simulink model "VCMGCM1962020b_v2"  (R2020b)
settings: Solver=FixedStepDiscrete  StartTime=0.0  StopTime=10.0  FixedStep=0.005  RelTol=1e-3  EnableMultiTasking=on
PreLoadFcn:
  | try, model_open; catch, disp('Error occurred while executing model pre-load callback: model_open.m'); disp('Please assure that the MATLAB working directory is set to the model directory before opening.'); end
InitFcn:
  | try, model_open; catch, end
undefined symbols (not defined in the file): Bridge, GCM, H, raptor_get_param_eval, raptor_get_safe_string, raptor_xcp_function
libraries: Blocks_lib x1165, Raptor_lib x665, simulink x62, VCM_lib x5
(part 3 of 23)

== system VCMGCM1962020b_v2/Fgnd/Actuators/CAN/CCS Interface ==
  Data : Inport
  Bus Creator : BusCreator  Inputs=1
  CCSEV_ChargeParameters1 : Subsystem
      mask help:
      | Example of how to set up a CAN message transmit.
      | 1. Copy this block into the main model.
      | 2. Disable/break library link.
      | 3. Underneath, set up CAN Tx Message block.
      | 4. For each field, connect a CANTxField block from the CAN block to the bus creator; adjust parameters as necessary.
      mask init:
      | [msgnam, msgbus] = CANBlockInit('Tx');
      mask Display: disp(['CAN Tx: Message\n' msgnam '\n' msgbus]);
  CCSEV_ChargeParameters2 : Subsystem
      mask help:
      | Example of how to set up a CAN message transmit.
      | 1. Copy this block into the main model.
      | 2. Disable/break library link.
      | 3. Underneath, set up CAN Tx Message block.
      | 4. For each field, connect a CANTxField block from the CAN block to the bus creator; adjust parameters as necessary.
      mask init:
      | [msgnam, msgbus] = CANBlockInit('Tx');
      mask Display: disp(['CAN Tx: Message\n' msgnam '\n' msgbus]);
  CCSEV_DC_ChargeInfo1 : Subsystem
      mask help:
      | Example of how to set up a CAN message transmit.
      | 1. Copy this block into the main model.
      | 2. Disable/break library link.
      | 3. Underneath, set up CAN Tx Message block.
      | 4. For each field, connect a CANTxField block from the CAN block to the bus creator; adjust parameters as necessary.
      mask init:
      | [msgnam, msgbus] = CANBlockInit('Tx');
      mask Display: disp(['CAN Tx: Message\n' msgnam '\n' msgbus]);
  Commands : Subsystem
  Header : Blocks_lib/Header  width=Portrait  addtext=''
  MsgName : Subsystem
      mask help:
      | Example of how to set up a CAN message transmit.
      | 1. Copy this block into the main model.
      | 2. Disable/break library link.
      | 3. Underneath, set up CAN Tx Message block.
      | 4. For each field, connect a CANTxField block from the CAN block to the bus creator; adjust parameters as necessary.
      mask init:
      | [msgnam, msgbus] = CANBlockInit('Tx');
      mask Display: disp(['CAN Tx: Message\n' msgnam '\n' msgbus]);
  Act : Outport  VectorParamsAs1DForOutWhenUnconnected=off
  wires:
  Commands/1(Cmds) -> Bus Creator/1, MsgName/2(Cmd), CCSEV_DC_ChargeInfo1/2(Cmd)
  Data/1 -> CCSEV_DC_ChargeInfo1/1(Data), CCSEV_ChargeParameters2/1(Data), CCSEV_ChargeParameters1/1(Data), MsgName/1(Data), Commands/1(Data)
  Bus Creator/1 -> Act/1  "CCS"

== system VCMGCM1962020b_v2/Fgnd/Actuators/CAN/Charger ==
  Data : Inport
  ChgrBMSA : Subsystem
      mask help:
      | Example of how to set up a CAN message transmit.
      | 1. Copy this block into the main model.
      | 2. Disable/break library link.
      | 3. Underneath, set up CAN Tx Message block.
      | 4. For each field, connect a CANTxField block from the CAN block to the bus creator; adjust parameters as necessary.
      mask init:
      | [msgnam, msgbus] = CANBlockInit('Tx');
      mask Display: disp(['CAN Tx: Message\n' msgnam '\n' msgbus]);
  Config Msgs : Subsystem  Commented=on
  Ground : Ground
  Header : Blocks_lib/Header  width=Portrait  addtext=''
  Act : Outport  VectorParamsAs1DForOutWhenUnconnected=off
  wires:
  Data/1 -> ChgrBMSA/1(Data)
  Ground/1 -> Act/1  "Chgr"

== system VCMGCM1962020b_v2/Fgnd/Actuators/CAN/DC//DC Converter ==
  Data : Inport
  Ground : Ground
  Header : Blocks_lib/Header  width=Portrait  addtext=''
  MsgName : Subsystem
      mask help:
      | Example of how to set up a CAN message transmit.
      | 1. Copy this block into the main model.
      | 2. Disable/break library link.
      | 3. Underneath, set up CAN Tx Message block.
      | 4. For each field, connect a CANTxField block from the CAN block to the bus creator; adjust parameters as necessary.
      mask init:
      | [msgnam, msgbus] = CANBlockInit('Tx');
      mask Display: disp(['CAN Tx: Message\n' msgnam '\n' msgbus]);
  Act : Outport  VectorParamsAs1DForOutWhenUnconnected=off
  wires:
  Ground/1 -> Act/1  "DCDC"
  Data/1 -> MsgName/1(Data)

== system VCMGCM1962020b_v2/Fgnd/Actuators/CAN/DC//DC Converter1 ==
  Data : Inport
  DCDCDCDC_Cmmd_0_16V : Subsystem
      mask help:
      | Example of how to set up a CAN message transmit.
      | 1. Copy this block into the main model.
      | 2. Disable/break library link.
      | 3. Underneath, set up CAN Tx Message block.
      | 4. For each field, connect a CANTxField block from the CAN block to the bus creator; adjust parameters as necessary.
      mask init:
      | [msgnam, msgbus] = CANBlockInit('Tx');
      mask Display: disp(['CAN Tx: Message\n' msgnam '\n' msgbus]);
  Ground : Ground
  Header : Blocks_lib/Header  width=Portrait  addtext=''
  Act : Outport  VectorParamsAs1DForOutWhenUnconnected=off
  wires:
  Ground/1 -> Act/1  "DCDC"
  Data/1 -> DCDCDCDC_Cmmd_0_16V/1(Data)

== system VCMGCM1962020b_v2/Fgnd/Actuators/CAN/Display ==
  Data : Inport
  DisplayHVES1_D2 : Subsystem
      mask help:
      | Example of how to set up a CAN message transmit.
      | 1. Copy this block into the main model.
      | 2. Disable/break library link.
      | 3. Underneath, set up CAN Tx Message block.
      | 4. For each field, connect a CANTxField block from the CAN block to the bus creator; adjust parameters as necessary.
      mask init:
      | [msgnam, msgbus] = CANBlockInit('Tx');
      mask Display: disp(['CAN Tx: Message\n' msgnam '\n' msgbus]);
  Ground : Ground
  Header : Blocks_lib/Header  width=Portrait  addtext=''
  Act : Outport  VectorParamsAs1DForOutWhenUnconnected=off
  wires:
  Ground/1 -> Act/1  "Dspl"
  Data/1 -> DisplayHVES1_D2/1(Data)

== system VCMGCM1962020b_v2/Fgnd/Actuators/CAN/Drive Inverter ==
  Data : Inport
  Bus Creator : BusCreator  Inputs=1
  Bus Selector : BusSelector  OutputSignals=Sensors.CAN.DrvInvtr.EM1.EM1MsgVld [Bool],Control.Mode.StartStop.RunMode [Bool]
  Bus Selector1 : BusSelector  OutputSignals=Sensors.CAN.DrvInvtr.EM1.EM1MsgVld [Bool],Control.DrvInvtr.DrvInvtrEnblReq [Bool]
  DrvInvtrNMT : Subsystem
      mask help:
      | Example of how to set up a CAN message transmit.
      | 1. Copy this block into the main model.
      | 2. Disable/break library link.
      | 3. Underneath, set up CAN Tx Message block.
      | 4. For each field, connect a CANTxField block from the CAN block to the bus creator; adjust parameters as necessary.
      mask init:
      | [msgnam, msgbus] = CANBlockInit('Tx');
      mask Display: disp(['CAN Tx: Message\n' msgnam '\n' msgbus]);
  DrvInvtrVCU1 : Subsystem
      mask help:
      | Example of how to set up a CAN message transmit.
      | 1. Copy this block into the main model.
      | 2. Disable/break library link.
      | 3. Underneath, set up CAN Tx Message block.
      | 4. For each field, connect a CANTxField block from the CAN block to the bus creator; adjust parameters as necessary.
      mask init:
      | [msgnam, msgbus] = CANBlockInit('Tx');
      mask Display: disp(['CAN Tx: Message\n' msgnam '\n' msgbus]);
  DrvInvtrVCU2 : Subsystem
      mask help:
      | Example of how to set up a CAN message transmit.
      | 1. Copy this block into the main model.
      | 2. Disable/break library link.
      | 3. Underneath, set up CAN Tx Message block.
      | 4. For each field, connect a CANTxField block from the CAN block to the bus creator; adjust parameters as necessary.
      mask init:
      | [msgnam, msgbus] = CANBlockInit('Tx');
      mask Display: disp(['CAN Tx: Message\n' msgnam '\n' msgbus]);
  Function-Call Subsystem : Subsystem  Commented=on  TreatAsAtomicUnit=on
  Ground1 : Ground
  Header : Blocks_lib/Header  width=Portrait  addtext=''
  Meas&Ovrd : Blocks_lib/Meas&Ovrd  nam='NMT_Step'  name_source=Parameter  view_as=Number  enum_struct={}  gain=1  min=-inf  max=inf  precision=''  units='nd'  help='Input valid'  group='Actuators | Inverter'
  Meas&Ovrd9 : Blocks_lib/Meas&Ovrd  nam='NMTLogicHVdetect'  name_source=Parameter  view_as=Number  enum_struct={}  gain=1  min=-inf  max=inf  precision=''  units='Bool'  help=''  group='Actuators | DrvInverter'
  NMT Sequence : Stateflow chart  TreatAsAtomicUnit=on
  NMT Trasition Command : Subsystem
      settings: OpenFcn=open_system(gcb,'force')
  State Transition Command1 : Subsystem  Commented=on
      settings: OpenFcn=open_system(gcb,'force')
  raptor_adjustment : Raptor_lib/Data Storage/raptor_adjustment  paramName='NMStateTrnsDly'  nameSource=Parameter  initValue=.1  dataType=double  storage=Calibration  calDispType=Number  calEnum={'False', 'True'}  calGain=samptime  calOffset=0.0  calMax=inf  calMin=-inf  calFormat='-1'  calUnit='sec'  calHelp='delay time formNMT message state change'  calAccess=1  calFunction="['Actuators | CAN |  DrvInvrtr']"  calDispHeaders=off  calColHeaders={'Col1' 'Col2' 'Col3'}  calRowHeaders={'Row1' 'Row2' 'Row3'}
      settings: SourceProductName=Raptor
  raptor_adjustment1 : Raptor_lib/Data Storage/raptor_adjustment  paramName='NMStateTrnsNoComTmOut'  nameSource=Parameter  initValue=.5  dataType=double  storage=Calibration  calDispType=Number  calEnum={'False', 'True'}  calGain=samptime  calOffset=0.0  calMax=inf  calMin=-inf  calFormat='-1'  calUnit='sec'  calHelp=' time to detect a No COmm condition with the Invrtr'  calAccess=1  calFunction="['Actuators | CAN |  DrvInvrtr']"  calDispHeaders=off  calColHeaders={'Col1' 'Col2' 'Col3'}  calRowHeaders={'Row1' 'Row2' 'Row3'}
      settings: SourceProductName=Raptor
  raptor_adjustment2 : Raptor_lib/Data Storage/raptor_adjustment  paramName='InvrtrAutoStartEnbled'  nameSource=Parameter  initValue=1  dataType=boolean  storage=Calibration  calDispType=Number  calEnum={'False', 'True'}  calGain=samptime  calOffset=0.0  calMax=inf  calMin=-inf  calFormat='-1'  calUnit='sec'  calHelp=' Bypass NMT logic when this is set to 1'  calAccess=1  calFunction="['Actuators | CAN |  DrvInvrtr']"  calDispHeaders=off  calColHeaders={'Col1' 'Col2' 'Col3'}  calRowHeaders={'Row1' 'Row2' 'Row3'}
      settings: SourceProductName=Raptor
  raptor_can_trigger : Raptor_lib/CAN/raptor_can_trigger  Commented=on  mailbox='DrvInvtrEM_BOOT'  inherited=0  alwaysEnabled=1  triggerPriority=0
      settings: SourceProductName=Raptor
  Act : Outport  VectorParamsAs1DForOutWhenUnconnected=off
  wires:
  NMT Trasition Command/1(State) -> DrvInvtrNMT/1(State), DrvInvtrVCU2/1(State), DrvInvtrVCU1/1(State)
  raptor_can_trigger/1 -> Function-Call Subsystem/Trigger
  Bus Selector/1 -> NMT Sequence/2(EMxRcved)  "<EM1MsgVld [Bool]>"
  raptor_adjustment/1 -> NMT Sequence/1(NMTStateDly)
  raptor_adjustment1/1 -> NMT Sequence/3(NoComTm)
  Meas&Ovrd9/1 -> NMT Sequence/4(HV_On)
  Bus Selector/2 -> NMT Sequence/5(RunMode)  "<RunMode [Bool]>"
  Ground1/1 -> Meas&Ovrd9/1
  Bus Selector1/1 -> NMT Sequence/6(EM1StateAct)  "<EM1MsgVld [Bool]>"
  Data/1 -> NMT Trasition Command/2(Data), DrvInvtrNMT/2(Data), DrvInvtrVCU1/2(Data), DrvInvtrVCU2/2(Data), Bus Selector1/1, Bus Selector/1
  Bus Selector1/2 -> NMT Sequence/7(InvrtrEnble)  "<DrvInvtrEnblReq [Bool]>"
  Bus Creator/1 -> Act/1  "DrvInvrtr"
  NMT Sequence/1(NMTStep) -> Bus Creator/1, Meas&Ovrd/1  "NMTStep"
  raptor_adjustment2/1 -> NMT Sequence/8(AutoStrEnbl)
  Meas&Ovrd/1 -> NMT Trasition Command/1(NMT_Step)

== system VCMGCM1962020b_v2/Fgnd/Actuators/CAN/Other ==
  Data : Inport
  A/C Compressor : Subsystem  mask{nam='ACC', bus='CAN1'}
      mask prompts: nam "Name"; bus "CAN Bus"
      mask Display: disp(['A/C Comp.: Mitsubishi EV36BNx\n' nam '\n' bus]);
  Bus Creator : BusCreator  Inputs=6
  Cooling Pump 1 : Subsystem  mask{nam='CoolPump1', bus='CAN1'}
      mask prompts: nam "Name"; bus "CAN Bus"
      mask Display: disp(['Water Pump: EMP WP29 (J1939)\n' nam '\n' bus]);
  Cooling Pump 2 : Subsystem  mask{nam='CoolPump2', bus='CAN1'}
      mask prompts: nam "Name"; bus "CAN Bus"
      mask Display: disp(['Water Pump: EMP WP29 (J1939)\n' nam '\n' bus]);
  Header : Blocks_lib/Header  width=Portrait  addtext=''
  Heater : Subsystem  mask{bus='CAN1'}
      mask prompts: bus "CAN Bus"
      mask Display: disp(['Heater: Mitsubishi EWH40Dx\n' bus]);
  MPDM : Subsystem  mask{nam='MPDM', bus='CAN1'}
      mask prompts: nam "Name"; bus "CAN Bus"
      mask Display: disp(['MPDM\n' nam '\n' bus]);
  Power Steering Pump Inverter : Subsystem  Commented=on  mask{nam='PSPInvtr', bus='CAN1'}
      mask prompts: nam "Name"; bus "CAN Bus"
      mask Display: disp(['Inverter: Sevcon HVLP-20\n' nam '\n' bus]);
  CAN : Outport  VectorParamsAs1DForOutWhenUnconnected=off
  wires:
  Bus Creator/1 -> CAN/1  "Other"
  Data/1 -> A/C Compressor/1(Data), Heater/1(Data), Cooling Pump 2/1(Data), MPDM/1(Data), Cooling Pump 1/1(Data), Power Steering Pump Inverter/1(Data)
  Power Steering Pump Inverter/1(Act) -> Bus Creator/1
  A/C Compressor/1(Act) -> Bus Creator/2
  Heater/1(Act) -> Bus Creator/3
  Cooling Pump 1/1(Act) -> Bus Creator/4
  MPDM/1(Act) -> Bus Creator/6
  Cooling Pump 2/1(Act) -> Bus Creator/5

== system VCMGCM1962020b_v2/Fgnd/Actuators/Command_G7/MsgTx ==
  Data : Inport
  Enable : EnablePort
  CANTxField : Blocks_lib/CANTxField  custom=off  custom_nam='---'  custom_units='---'
  Header : Blocks_lib/Header  width=Landscape  addtext=''
  raptor_can_txmsg : Raptor_lib/CAN/raptor_can_txmsg  canDefinition=struct('dbcFile', 'EPAS_dbc_file_rev2.0.dbc','message', 'Command_G7','comment', '','signals', {{'Cmmd_mode','Variable_1','Variable_2'}},'enabled', [ 1 0 0;],'scaled', [ 1 1 1;],'canBus', '''CAN1''','messageID', [ 419406831;],'idMask', [ 536870911;],'payloadMask', [],'payloadValue', [],'period', [ 100;],'mailbox', '''''','queueSize', [ 1;],'label', [ 1;],'ver', [ 2;],'showID', [ 0;],'showRaw', [ 0;],'fill', [ 0;],'editID', [ 0;],'signalOrder', [ 3;],'signalAscDes', [ 1;])  canBus='CAN1'  queueSize=1  payloadMask=[]  payloadValue=[]  period=100  showID=0  label=1  idMask=hex2dec('1FFFFFFF')  fill=0  id=419406831  showRaw=0  signalOrder=3  signalInfo={{struct('Name', 'Cmmd_mode','Startbit', [ 0;],'SignalSize', [ 8;],'ByteOrder', 'LittleEndian','ValueType', 'UNSIGNED','Class', 'uint8','Signed', [ 0;],'Factor', [ 1;],'Offset', [ 0;],'Min', [ 0;],'Max', [ 5;],'Units', '','Comment', '','StartBit', [ 0;]),struct('Name', 'Variable_1','Startbit', [ 0;],'SignalSize', [ 32;],'ByteOrder', 'LittleEndian','ValueType', 'UNSIGNED','Class', 'uint32','Signed', [ 0;],'Factor', [ 3.8147e-06;],'Offset', [ 0;],'Min', [ -8192;],'Max', [ 8192;],'Units', '','Comment', '','StartBit', [ 16;]),struct('Name', 'Variable_2','Startbit', [ 0;],'SignalSize', [ 16;],'ByteOrder', 'LittleEndian','ValueType', 'UNSIGNED','Class', 'uint16','Signed', [ 0;],'Factor', [ 0.0039063;],'Offset', [ 0;],'Min', [ -255;],'Max', [ 255;],'Units', '','Comment', '','StartBit', [ 48;])}}
      settings: SourceProductName=Raptor
  wires:
  CANTxField/1 -> raptor_can_txmsg/1  "Cmmd_mode"
  Data/1 -> ?

== system VCMGCM1962020b_v2/Fgnd/Actuators/FMWS/MCU_130h ==
  Data : Inport
  CANTxMsgEnbl : Blocks_lib/CANTxMsgEnbl  custom=off  custom_nam=[nam '---']  msgnam=MCU_130h
  FMWS Enbl : Subsystem
  Header : Blocks_lib/Header  width=Portrait  addtext=''
  MsgTx : Subsystem
  wires:
  CANTxMsgEnbl/1 -> MsgTx/Enable
  Data/1 -> MsgTx/1(Data), FMWS Enbl/1(In1)
  FMWS Enbl/1(Out1) -> CANTxMsgEnbl/1

== system VCMGCM1962020b_v2/Fgnd/Actuators/FMWS/MCU_131h ==
  Data : Inport
  Bus Selector : BusSelector  OutputSignals=Control.Mode.StartStop.ModWake [Bool]
  CANTxMsgEnbl : Blocks_lib/CANTxMsgEnbl  custom=off  custom_nam=[nam '---']  msgnam=MCU_131h
  Header : Blocks_lib/Header  width=Portrait  addtext=''
  MsgTx : Subsystem
  wires:
  Data/1 -> MsgTx/1(Data), Bus Selector/1
  CANTxMsgEnbl/1 -> MsgTx/Enable
  Bus Selector/1 -> CANTxMsgEnbl/1  "<ModWake [Bool]>"

== system VCMGCM1962020b_v2/Fgnd/Actuators/FMWS_J1939/CCVS ==
  Data : Inport
  Bus Selector : BusSelector  OutputSignals=Control.Mode.StartStop.ModWake [Bool]
  CANTxMsgEnbl : Blocks_lib/CANTxMsgEnbl  custom=off  custom_nam=[nam '---']  msgnam=CCVS
  Header : Blocks_lib/Header  width=Portrait  addtext=''
  MsgTx : Subsystem
  wires:
  Data/1 -> MsgTx/1(Data), Bus Selector/1
  CANTxMsgEnbl/1 -> MsgTx/Enable
  Bus Selector/1 -> CANTxMsgEnbl/1  "<ModWake [Bool]>"

== system VCMGCM1962020b_v2/Fgnd/Actuators/FMWS_J1939/ETC2 ==
  Data : Inport
  Bus Selector : BusSelector  OutputSignals=Control.Mode.StartStop.ModWake [Bool]
  CANTxMsgEnbl : Blocks_lib/CANTxMsgEnbl  custom=off  custom_nam=[nam '---']  msgnam=ETC2
  Header : Blocks_lib/Header  width=Portrait  addtext=''
  MsgTx : Subsystem
  wires:
  Bus Selector/1 -> CANTxMsgEnbl/1  "<ModWake [Bool]>"
  CANTxMsgEnbl/1 -> MsgTx/Enable
  Data/1 -> Bus Selector/1, MsgTx/1(Data)

== system VCMGCM1962020b_v2/Fgnd/Control/Drive Inverter/Inverter Enable Request ==
  Data : Inport
  Bus Selector : BusSelector  OutputSignals=Control.Mode.StartStop.RunMode [Bool],Control.Mode.PRNDMode [enum]
  Bus Selector1 : BusSelector  OutputSignals=VirtualSensors.Chgr.ChgPlugState [enum]
  CmprTo : Blocks_lib/CmprTo  op===  val='Drv'  enum=EnumLst.PRNDMode
  CmprTo1 : Blocks_lib/CmprTo  op===  val='Rev'  enum=EnumLst.PRNDMode
  CmprTo2 : Blocks_lib/CmprTo  op===  val='Disconnected'  enum=EnumLst.ChgPlugState
  Header : Blocks_lib/Header  width=Portrait  addtext=''
  Logical Operator : Logic  Inputs=5  OutDataTypeStr=boolean
  Logical Operator1 : Logic  Operator=OR  OutDataTypeStr=boolean
  Logical Operator2 : Logic  Operator=NOT  Inputs=1  OutDataTypeStr=boolean
  raptor_adjustment : Raptor_lib/Data Storage/raptor_adjustment  paramName='DrvInvtrEnblReqEnbl'  nameSource=Parameter  initValue=0  dataType=boolean  storage=Calibration  calDispType=Number  calEnum={'False', 'True'}  calGain=1  calOffset=0  calMax=inf  calMin=-inf  calFormat=''  calUnit='Bool'  calHelp='Drive inverter enable request enable'  calAccess=1  calFunction=group  calDispHeaders=off  calColHeaders={'Col1' 'Col2' 'Col3'}  calRowHeaders={'Row1' 'Row2' 'Row3'}
      settings: SourceProductName=Raptor
  raptor_fault_action : Raptor_lib/Faults/raptor_fault_action  actionName='DrvInvtrDsbl'  calVisible=off  calAccess=1  calFunction='System | FaultManager | FaultAction'
      settings: SourceProductName=Raptor
  raptor_measurement : Raptor_lib/Data Storage/raptor_measurement  paramName='DrvInvtrEnblReq'  nameSource=Parameter  calDispType=Number  calEnum={'False', 'True'}  calGain=1.0  calOffset=0.0  calMax=inf  calMin=-inf  calFormat='-1'  calUnit='Bool'  calHelp=''  calAccess=1  calFunction=group  calVisible=on
      settings: SourceProductName=Raptor
  Bool : Outport  VectorParamsAs1DForOutWhenUnconnected=off
  wires:
  raptor_adjustment/1 -> Logical Operator/1
  raptor_fault_action/1 -> Logical Operator2/1
  Logical Operator/1 -> raptor_measurement/1, Bool/1
  CmprTo2/1 -> Logical Operator/4
  Bus Selector1/1 -> CmprTo2/1  "<ChgPlugState [enum]>"
  CmprTo/1 -> Logical Operator1/1
  Logical Operator2/1 -> Logical Operator/5
  CmprTo1/1 -> Logical Operator1/2
  Bus Selector/2 -> CmprTo1/1, CmprTo/1  "<PRNDMode [enum]>"
  Logical Operator1/1 -> Logical Operator/3
  Data/1 -> Bus Selector/1, Bus Selector1/1
  Bus Selector/1 -> Logical Operator/2  "<RunMode [Bool]>"

== system VCMGCM1962020b_v2/Fgnd/Control/Drive Inverter/Motor Torque Request ==
  Data : Inport
  EnblReq : Inport  Port=2
  Bus Creator : BusCreator  Inputs=3
  Current/Torque Split : Subsystem
  Driver Torque Request : Subsystem  mask{group=[group ' | Driver Torque Request']}
  Header : Blocks_lib/Header  width=Portrait  addtext=''
  Inverter/Motor Limit & Request : Subsystem  mask{invtrnam='DrvInvtr', mtrnam='DrvMtr', group=group}
      mask prompts: invtrnam "Inverter Name"; mtrnam "Motor Name"
      mask init:
      | cb = gcb;
      | 
      | % --- Name Line
      | NameLine([cb '/Inverter Current Limit/BusCreator'], 'Inport(1)', [invtrnam 'MCL [A]']);
      | NameLine([cb '/Inverter Current Limit/BusCreator'], 'Inport(2)', [invtrnam 'GCL [A]']);
      | NameLine([cb '/BusCreator'], 'Inport(2)', [mtrnam 'TrqLim [Nm]']);
      | NameLine([cb '/BusCreator'], 'Inport(3)', [mtrnam 'TrqReq [Nm]']);
      | NameLine([cb '/BusCreator'], 'Outport(1)', invtrnam);
      mask Display: disp(['Inverter/Motor\nLimit & Request\n(' invtrnam ', ' mtrnam ')']);
  MtrTrqReq : Outport  VectorParamsAs1DForOutWhenUnconnected=off
  wires:
  Driver Torque Request/1(TrqReq) -> Current/Torque Split/2(TrqReq), Bus Creator/1
  Bus Creator/1 -> MtrTrqReq/1  "MtrTrqReq"
  Data/1 -> Driver Torque Request/1(Data), Inverter/Motor Limit & Request/1(Data), Current/Torque Split/1(Data)
  Current/Torque Split/1(Split) -> Bus Creator/2, Inverter/Motor Limit & Request/3(Split)
  Inverter/Motor Limit & Request/1(InvtrMtr) -> Bus Creator/3
  EnblReq/1 -> Inverter/Motor Limit & Request/2(EnblReq)

== system VCMGCM1962020b_v2/Fgnd/Control/Modes/PRND Mode ==
  note: This stateflow chart was used with FMWS and dipay.
      | Can be removed if no longer usefull.
  Data : Inport
  AllowShiftFromPark : Subsystem
  Bus Selector : BusSelector  OutputSignals=Control.Mode.StartStop.RunMode [Bool],VirtualSensors.Spd.VehSpd [kph]
  Bus Selector1 : BusSelector  OutputSignals=Control.Mode.StartStop.ChgMode [Bool]
  Header : Blocks_lib/Header  width=Portrait  addtext=''
  Meas&Ovrd : Blocks_lib/Meas&Ovrd  nam='PRNDMode'  name_source=Parameter  view_as=Enumeration  enum_struct=EnumLst.PRNDMode  gain=1  min=-inf  max=inf  precision=''  units='enum'  help='PRND mode'  group=group
  PRND : Subsystem
  PRND Mode : Stateflow chart  TreatAsAtomicUnit=on
  PRND_Act : Stateflow chart  TreatAsAtomicUnit=on
  PRND_FMWS : Stateflow chart  TreatAsAtomicUnit=on
  raptor_adjustment : Raptor_lib/Data Storage/raptor_adjustment  paramName='PRNDModeVehSpdZeroThr'  nameSource=Parameter  initValue=0  dataType=double  storage=Calibration  calDispType=Number  calEnum={'Disabled', 'Enabled'}  calGain=1  calOffset=0  calMax=inf  calMin=-inf  calFormat=''  calUnit='kph'  calHelp='PRND mode vehicle speed zero threshold'  calAccess=1  calFunction=group  calDispHeaders=off  calColHeaders={'Col1' 'Col2' 'Col3'}  calRowHeaders={'Row1' 'Row2' 'Row3'}
      settings: SourceProductName=Raptor
  raptor_adjustment1 : Raptor_lib/Data Storage/raptor_adjustment  paramName='PRNDModeVehSpdLoThr'  nameSource=Parameter  initValue=0  dataType=double  storage=Calibration  calDispType=Number  calEnum={'Disabled', 'Enabled'}  calGain=1  calOffset=0  calMax=inf  calMin=-inf  calFormat=''  calUnit='kph'  calHelp='PRND mode vehicle speed low threshold'  calAccess=1  calFunction=group  calDispHeaders=off  calColHeaders={'Col1' 'Col2' 'Col3'}  calRowHeaders={'Row1' 'Row2' 'Row3'}
      settings: SourceProductName=Raptor
  enum : Outport  VectorParamsAs1DForOutWhenUnconnected=off
  enum1 : Outport  Port=2  VectorParamsAs1DForOutWhenUnconnected=off
  enum2 : Outport  Port=3  VectorParamsAs1DForOutWhenUnconnected=off
  wires:
  PRND Mode/1(PRNDMode) -> PRND_FMWS/1(PRND_In), PRND_Act/1(PRND_In), Meas&Ovrd/1
  raptor_adjustment/1 -> PRND Mode/8(SpdZeroThr)
  raptor_adjustment1/1 -> PRND Mode/9(SpdLoThr)
  Bus Selector/1 -> PRND Mode/6(RunMode)  "<RunMode [Bool]>"
  AllowShiftFromPark/1(Bool) -> PRND Mode/5(AllowShiftFromPark)
  Meas&Ovrd/1 -> enum/1
  Bus Selector/2 -> PRND Mode/7(Spd)  "<VehSpd [kph]>"
  Data/1 -> Bus Selector1/1, Bus Selector/1, AllowShiftFromPark/1(Data), PRND/1(Data)
  PRND/1(P) -> PRND Mode/1(Park)
  PRND/2(R) -> PRND Mode/2(Reverse)
  PRND/3(N) -> PRND Mode/3(Neutral)
  PRND/4(D) -> PRND Mode/4(Drive)
  PRND_Act/1(PRND_Act_Out) -> enum1/1
  Bus Selector1/1 -> PRND Mode/10(ChgMode)  "<ChgMode [Bool]>"
  PRND_FMWS/1(PRND_Act_Out) -> enum2/1

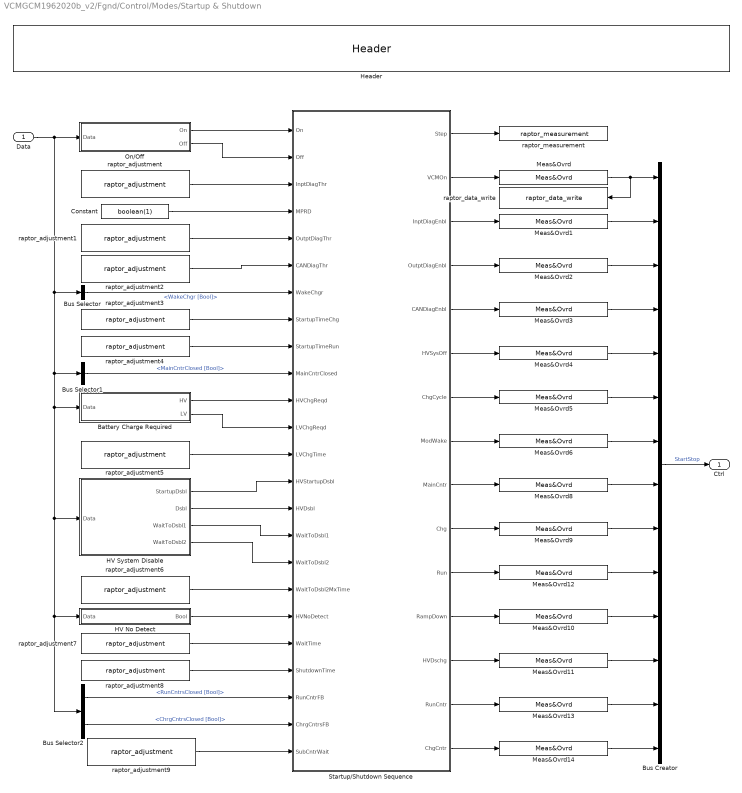
== system VCMGCM1962020b_v2/Fgnd/Control/Modes/Startup & Shutdown ==
  Data : Inport
  Battery Charge Required : Subsystem
  Bus Creator : BusCreator  Inputs=14
  Bus Selector : BusSelector  OutputSignals=Sensors.Sensors.Volt.WakeChgr.WakeChgr [Bool]
  Bus Selector1 : BusSelector  OutputSignals=VirtualSensors.PDU.MainCntrClosed [Bool]
  Bus Selector2 : BusSelector  OutputSignals=Control.PDU.PDUCntrs.RunCntrsClosed [Bool],Control.PDU.PDUCntrs.ChrgCntrsClosed [Bool]
  Constant : Constant  Value=boolean(1)
  HV No Detect : Subsystem
  HV System Disable : Subsystem
  Header : Blocks_lib/Header  width=Portrait  addtext=''
  Meas&Ovrd : Blocks_lib/Meas&Ovrd  nam='VCMOn'  name_source=Parameter  view_as=Number  enum_struct={}  gain=1  min=-inf  max=inf  precision=''  units='Bool'  help='Module to be powered on or off'  group=group
  Meas&Ovrd1 : Blocks_lib/Meas&Ovrd  nam='InptDiagEnbl'  name_source=Parameter  view_as=Number  enum_struct={}  gain=1  min=-inf  max=inf  precision=''  units='Bool'  help='Input diagnostics enabled'  group=group
  Meas&Ovrd10 : Blocks_lib/Meas&Ovrd  nam='RampDown'  name_source=Parameter  view_as=Number  enum_struct={}  gain=1  min=-inf  max=inf  precision=''  units='Bool'  help='Ramp down'  group=group
  Meas&Ovrd11 : Blocks_lib/Meas&Ovrd  nam='HVDschg'  name_source=Parameter  view_as=Number  enum_struct={}  gain=1  min=-inf  max=inf  precision=''  units='Bool'  help='High-voltage discharge'  group=group
  Meas&Ovrd12 : Blocks_lib/Meas&Ovrd  nam='RunMode'  name_source=Parameter  view_as=Number  enum_struct={}  gain=1  min=-inf  max=inf  precision=''  units='Bool'  help='Run mode'  group=group
  Meas&Ovrd13 : Blocks_lib/Meas&Ovrd  nam='RunCntr'  name_source=Parameter  view_as=Number  enum_struct={}  gain=1  min=-inf  max=inf  precision=''  units='Bool'  help='Sub Syst Cntr Cmd'  group=group
  Meas&Ovrd14 : Blocks_lib/Meas&Ovrd  nam='ChgCntr'  name_source=Parameter  view_as=Number  enum_struct={}  gain=1  min=-inf  max=inf  precision=''  units='Bool'  help='Charger Contactor Cmd'  group=group
  Meas&Ovrd2 : Blocks_lib/Meas&Ovrd  nam='OutptDiagEnbl'  name_source=Parameter  view_as=Number  enum_struct={}  gain=1  min=-inf  max=inf  precision=''  units='Bool'  help='Output diagnostics enabled'  group=group
  Meas&Ovrd3 : Blocks_lib/Meas&Ovrd  nam='CANDiagEnbl'  name_source=Parameter  view_as=Number  enum_struct={}  gain=1  min=-inf  max=inf  precision=''  units='Bool'  help='CAN diagnostics enabled'  group=group
  Meas&Ovrd4 : Blocks_lib/Meas&Ovrd  nam='HVSysOff'  name_source=Parameter  view_as=Number  enum_struct={}  gain=1  min=-inf  max=inf  precision=''  units='Bool'  help='High-voltage system off'  group=group
  Meas&Ovrd5 : Blocks_lib/Meas&Ovrd  nam='ChgCycle'  name_source=Parameter  view_as=Number  enum_struct={}  gain=1  min=-inf  max=inf  precision=''  units='Bool'  help='Charge cycle'  group=group
  Meas&Ovrd6 : Blocks_lib/Meas&Ovrd  nam='ModWake'  name_source=Parameter  view_as=Number  enum_struct={}  gain=1  min=-inf  max=inf  precision=''  units='Bool'  help='Module wake-up'  group=group
  Meas&Ovrd8 : Blocks_lib/Meas&Ovrd  nam='MainCntrReq'  name_source=Parameter  view_as=Number  enum_struct={}  gain=1  min=-inf  max=inf  precision=''  units='Bool'  help='Main contactor request'  group=group
  Meas&Ovrd9 : Blocks_lib/Meas&Ovrd  nam='ChgMode'  name_source=Parameter  view_as=Number  enum_struct={}  gain=1  min=-inf  max=inf  precision=''  units='Bool'  help='Charge mode'  group=group
  On/Off : Subsystem
  Startup/Shutdown Sequence : Stateflow chart  TreatAsAtomicUnit=on
  raptor_adjustment : Raptor_lib/Data Storage/raptor_adjustment  paramName='InptDiagEnblTimeThr'  nameSource=Parameter  initValue=0  dataType=uint16  storage=Calibration  calDispType=Number  calEnum={'False', 'True'}  calGain=samptime  calOffset=0.0  calMax=inf  calMin=-inf  calFormat='0.3'  calUnit='sec'  calHelp='Input diagnostics enable time (after VCM on)'  calAccess=1  calFunction=group  calDispHeaders=off  calColHeaders={'Col1' 'Col2' 'Col3'}  calRowHeaders={'Row1' 'Row2' 'Row3'}
      settings: SourceProductName=Raptor
  raptor_adjustment1 : Raptor_lib/Data Storage/raptor_adjustment  paramName='OutptDiagEnblTimeThr'  nameSource=Parameter  initValue=0  dataType=uint16  storage=Calibration  calDispType=Number  calEnum={'False', 'True'}  calGain=samptime  calOffset=0.0  calMax=inf  calMin=-inf  calFormat='0.3'  calUnit='sec'  calHelp='Output diagnostics enable time (after main power relay closed)'  calAccess=1  calFunction=group  calDispHeaders=off  calColHeaders={'Col1' 'Col2' 'Col3'}  calRowHeaders={'Row1' 'Row2' 'Row3'}
      settings: SourceProductName=Raptor
  raptor_adjustment2 : Raptor_lib/Data Storage/raptor_adjustment  paramName='CANDiagEnblTimeThr'  nameSource=Parameter  initValue=0  dataType=uint16  storage=Calibration  calDispType=Number  calEnum={'Disabled', 'Enabled'}  calGain=samptime  calOffset=0  calMax=inf  calMin=-inf  calFormat='0.3'  calUnit='sec'  calHelp='CAN diagnostics enable time (after VCM on)'  calAccess=1  calFunction=group  calDispHeaders=off  calColHeaders={'Col1' 'Col2' 'Col3'}  calRowHeaders={'Row1' 'Row2' 'Row3'}
      settings: SourceProductName=Raptor
  raptor_adjustment3 : Raptor_lib/Data Storage/raptor_adjustment  paramName='ModStartupTimeChg'  nameSource=Parameter  initValue=0  dataType=uint16  storage=Calibration  calDispType=Number  calEnum={'False', 'True'}  calGain=samptime  calOffset=0.0  calMax=inf  calMin=-inf  calFormat='0.3'  calUnit='sec'  calHelp='Module startup time (before charge mode)'  calAccess=1  calFunction=group  calDispHeaders=off  calColHeaders={'Col1' 'Col2' 'Col3'}  calRowHeaders={'Row1' 'Row2' 'Row3'}
      settings: SourceProductName=Raptor
  raptor_adjustment4 : Raptor_lib/Data Storage/raptor_adjustment  paramName='ModStartupTimeRun'  nameSource=Parameter  initValue=0  dataType=uint16  storage=Calibration  calDispType=Number  calEnum={'False', 'True'}  calGain=samptime  calOffset=0.0  calMax=inf  calMin=-inf  calFormat='0.3'  calUnit='sec'  calHelp='Module startup time (before run mode)'  calAccess=1  calFunction=group  calDispHeaders=off  calColHeaders={'Col1' 'Col2' 'Col3'}  calRowHeaders={'Row1' 'Row2' 'Row3'}
      settings: SourceProductName=Raptor
  raptor_adjustment5 : Raptor_lib/Data Storage/raptor_adjustment  paramName='LVBattChgTime'  nameSource=Parameter  initValue=0  dataType=uint32  storage=Calibration  calDispType=Number  calEnum={'False', 'True'}  calGain=samptime  calOffset=0.0  calMax=inf  calMin=-inf  calFormat='0.3'  calUnit='sec'  calHelp='Low-voltage battery charge time'  calAccess=1  calFunction=group  calDispHeaders=off  calColHeaders={'Col1' 'Col2' 'Col3'}  calRowHeaders={'Row1' 'Row2' 'Row3'}
      settings: SourceProductName=Raptor
  raptor_adjustment6 : Raptor_lib/Data Storage/raptor_adjustment  paramName='HVSysWaitToDsbl2MxTime'  nameSource=Parameter  initValue=0  dataType=uint32  storage=Calibration  calDispType=Number  calEnum={'False', 'True'}  calGain=samptime  calOffset=0.0  calMax=inf  calMin=-inf  calFormat='0.3'  calUnit='sec'  calHelp='High-voltage system wait to disable (due to battery current) maximum time'  calAccess=1  calFunction=group  calDispHeaders=off  calColHeaders={'Col1' 'Col2' 'Col3'}  calRowHeaders={'Row1' 'Row2' 'Row3'}
      settings: SourceProductName=Raptor
  raptor_adjustment7 : Raptor_lib/Data Storage/raptor_adjustment  paramName='BattChgWaitTime'  nameSource=Parameter  initValue=0  dataType=uint32  storage=Calibration  calDispType=Number  calEnum={'False', 'True'}  calGain=samptime  calOffset=0.0  calMax=inf  calMin=-inf  calFormat='0.3'  calUnit='sec'  calHelp='Battery charge wait time (between charge attempts after charge completed)'  calAccess=1  calFunction=group  calDispHeaders=off  calColHeaders={'Col1' 'Col2' 'Col3'}  calRowHeaders={'Row1' 'Row2' 'Row3'}
      settings: SourceProductName=Raptor
  raptor_adjustment8 : Raptor_lib/Data Storage/raptor_adjustment  paramName='ModShutdownTime'  nameSource=Parameter  initValue=0  dataType=uint16  storage=Calibration  calDispType=Number  calEnum={'False', 'True'}  calGain=samptime  calOffset=0.0  calMax=inf  calMin=-inf  calFormat='0.3'  calUnit='sec'  calHelp='Module shutdown time'  calAccess=1  calFunction=group  calDispHeaders=off  calColHeaders={'Col1' 'Col2' 'Col3'}  calRowHeaders={'Row1' 'Row2' 'Row3'}
      settings: SourceProductName=Raptor
  raptor_adjustment9 : Raptor_lib/Data Storage/raptor_adjustment  paramName='CntrSubWaitTime'  nameSource=Parameter  initValue=1  dataType=uint32  storage=Calibration  calDispType=Number  calEnum={'False', 'True'}  calGain=samptime  calOffset=0.0  calMax=inf  calMin=-inf  calFormat='0.3'  calUnit='sec'  calHelp='Delay time before initiating Main cont cmd '  calAccess=1  calFunction=group  calDispHeaders=off  calColHeaders={'Col1' 'Col2' 'Col3'}  calRowHeaders={'Row1' 'Row2' 'Row3'}
      settings: SourceProductName=Raptor
  raptor_data_write : Raptor_lib/Data Storage/raptor_data_write  dataName='KeepModuleOn'  dataShape=Scalar  idxSource=Write Entire Vector/Matrix  idxRow=1  idxCol=1
      settings: SourceProductName=Raptor
  raptor_measurement : Raptor_lib/Data Storage/raptor_measurement  paramName='StartupShutdownStep'  nameSource=Parameter  calDispType=Number  calEnum={}  calGain=1.0  calOffset=0.0  calMax=inf  calMin=-inf  calFormat='-1'  calUnit=''  calHelp='Startup/shutdown step'  calAccess=1  calFunction=group  calVisible=on
      settings: SourceProductName=Raptor
  Ctrl : Outport  VectorParamsAs1DForOutWhenUnconnected=off
  wires:
  Bus Selector1/1 -> Startup/Shutdown Sequence/10(MainCntrClosed)  "<MainCntrClosed [Bool]>"
  Startup/Shutdown Sequence/5(CANDiagEnbl) -> Meas&Ovrd3/1
  Startup/Shutdown Sequence/4(OutptDiagEnbl) -> Meas&Ovrd2/1
  Startup/Shutdown Sequence/3(InptDiagEnbl) -> Meas&Ovrd1/1
  Meas&Ovrd/1 -> raptor_data_write/1, Bus Creator/1
  Startup/Shutdown Sequence/2(VCMOn) -> Meas&Ovrd/1
  Startup/Shutdown Sequence/11(Run) -> Meas&Ovrd12/1
  Startup/Shutdown Sequence/10(Chg) -> Meas&Ovrd9/1
  Startup/Shutdown Sequence/9(MainCntr) -> Meas&Ovrd8/1
  Startup/Shutdown Sequence/12(RampDown) -> Meas&Ovrd10/1
  Startup/Shutdown Sequence/13(HVDschg) -> Meas&Ovrd11/1
  Startup/Shutdown Sequence/8(ModWake) -> Meas&Ovrd6/1
  Startup/Shutdown Sequence/7(ChgCycle) -> Meas&Ovrd5/1
  raptor_adjustment4/1 -> Startup/Shutdown Sequence/9(StartupTimeRun)
  Data/1 -> On/Off/1(Data), Bus Selector2/1, HV No Detect/1(Data), HV System Disable/1(Data), Battery Charge Required/1(Data), Bus Selector1/1, Bus Selector/1
  raptor_adjustment1/1 -> Startup/Shutdown Sequence/5(OutptDiagThr)
  raptor_adjustment2/1 -> Startup/Shutdown Sequence/6(CANDiagThr)
  raptor_adjustment7/1 -> Startup/Shutdown Sequence/20(WaitTime)
  raptor_adjustment/1 -> Startup/Shutdown Sequence/3(InptDiagThr)
  Battery Charge Required/1(HV) -> Startup/Shutdown Sequence/11(HVChgReqd)
  Constant/1 -> Startup/Shutdown Sequence/4(MPRD)
  On/Off/1(On) -> Startup/Shutdown Sequence/1(On)
  raptor_adjustment5/1 -> Startup/Shutdown Sequence/13(LVChgTime)
  Bus Selector/1 -> Startup/Shutdown Sequence/7(WakeChgr)  "<WakeChgr [Bool]>"
  HV No Detect/1(Bool) -> Startup/Shutdown Sequence/19(HVNoDetect)
  raptor_adjustment8/1 -> Startup/Shutdown Sequence/21(ShutdownTime)
  raptor_adjustment6/1 -> Startup/Shutdown Sequence/18(WaitToDsbl2MxTime)
  raptor_adjustment3/1 -> Startup/Shutdown Sequence/8(StartupTimeChg)
  Startup/Shutdown Sequence/1(Step) -> raptor_measurement/1
  Bus Creator/1 -> Ctrl/1  "StartStop"
  Startup/Shutdown Sequence/6(HVSysOff) -> Meas&Ovrd4/1
  Meas&Ovrd2/1 -> Bus Creator/3
  Meas&Ovrd1/1 -> Bus Creator/2
  Meas&Ovrd3/1 -> Bus Creator/4
  Meas&Ovrd4/1 -> Bus Creator/5
  Meas&Ovrd5/1 -> Bus Creator/6
  Meas&Ovrd6/1 -> Bus Creator/7
  Meas&Ovrd8/1 -> Bus Creator/8
  Meas&Ovrd9/1 -> Bus Creator/9
  Meas&Ovrd12/1 -> Bus Creator/10
  Meas&Ovrd10/1 -> Bus Creator/11
  Meas&Ovrd11/1 -> Bus Creator/12
  HV System Disable/1(StartupDsbl) -> Startup/Shutdown Sequence/14(HVStartupDsbl)
  HV System Disable/2(Dsbl) -> Startup/Shutdown Sequence/15(HVDsbl)
  HV System Disable/3(WaitToDsbl1) -> Startup/Shutdown Sequence/16(WaitToDsbl1)
  HV System Disable/4(WaitToDsbl2) -> Startup/Shutdown Sequence/17(WaitToDsbl2)
  On/Off/2(Off) -> Startup/Shutdown Sequence/2(Off)
  Battery Charge Required/2(LV) -> Startup/Shutdown Sequence/12(LVChgReqd)
  Bus Selector2/1 -> Startup/Shutdown Sequence/22(RunCntrFB)  "<RunCntrsClosed [Bool]>"
  raptor_adjustment9/1 -> Startup/Shutdown Sequence/24(SubCntrWait)
  Startup/Shutdown Sequence/14(RunCntr) -> Meas&Ovrd13/1
  Startup/Shutdown Sequence/15(ChgCntr) -> Meas&Ovrd14/1
  Meas&Ovrd13/1 -> Bus Creator/13
  Meas&Ovrd14/1 -> Bus Creator/14
  Bus Selector2/2 -> Startup/Shutdown Sequence/23(ChrgCntrsFB)  "<ChrgCntrsClosed [Bool]>"

== system VCMGCM1962020b_v2/Fgnd/Control/Other/A//C Compressor ==
  Data : Inport
  Bus Creator : BusCreator  Inputs=2
  Bus Selector1 : BusSelector  OutputSignals=Control.Mode.StartStop.ChgMode [Bool],Control.Mode.StartStop.RunMode [Bool]
  Bus Selector2 : BusSelector  OutputSignals=VirtualSensors.Other.ACCReq [Bool]
  Bus Selector3 : BusSelector  OutputSignals=VirtualSensors.Other.ACPress [kPa]
  Bus Selector4 : BusSelector  OutputSignals=VirtualSensors.Other.ACEvapTemp [degC]
  Header : Blocks_lib/Header  width=Portrait  addtext=''
  Logical Operator : Logic  Inputs=5  OutDataTypeStr=boolean
  Logical Operator1 : Logic  Operator=OR  OutDataTypeStr=boolean
  RelOp(w/Hyst) : Blocks_lib/RelOp(w//Hyst)  relop=<=
  RelOp(w/Hyst)1 : Blocks_lib/RelOp(w//Hyst)  relop=>=
  Speed Request : Subsystem
  raptor_adjustment : Raptor_lib/Data Storage/raptor_adjustment  paramName='ACCEnblReqEnbl'  nameSource=Parameter  initValue=0  dataType=boolean  storage=Calibration  calDispType=Number  calEnum={'False', 'True'}  calGain=1  calOffset=0  calMax=inf  calMin=-inf  calFormat=''  calUnit='Bool'  calHelp='A/C compressor enable request enable'  calAccess=1  calFunction='Control | AC Compressor'  calDispHeaders=off  calColHeaders={'Col1' 'Col2' 'Col3'}  calRowHeaders={'Row1' 'Row2' 'Row3'}
      settings: SourceProductName=Raptor
  raptor_adjustment1 : Raptor_lib/Data Storage/raptor_adjustment  paramName='ACCEnblACPressThr'  nameSource=Parameter  initValue=[0 0]  dataType=double  storage=Calibration  calDispType=Number  calEnum={'False', 'True'}  calGain=1.0  calOffset=0.0  calMax=inf  calMin=-inf  calFormat=''  calUnit='kPa'  calHelp='A/C compressor enable threshold (on A/C pressure)'  calAccess=1  calFunction='Control | AC Compressor'  calDispHeaders=off  calColHeaders={'Col1' 'Col2' 'Col3'}  calRowHeaders={'Row1' 'Row2' 'Row3'}
      settings: SourceProductName=Raptor
  raptor_adjustment2 : Raptor_lib/Data Storage/raptor_adjustment  paramName='ACCEnblEvapTempThr'  nameSource=Parameter  initValue=[0 0]  dataType=double  storage=Calibration  calDispType=Number  calEnum={'False', 'True'}  calGain=1.0  calOffset=0.0  calMax=inf  calMin=-inf  calFormat=''  calUnit='degC'  calHelp='A/C compressor enable threshold (on A/C evaporator temperature)'  calAccess=1  calFunction='Control | AC Compressor'  calDispHeaders=off  calColHeaders={'Col1' 'Col2' 'Col3'}  calRowHeaders={'Row1' 'Row2' 'Row3'}
      settings: SourceProductName=Raptor
  Ctrl : Outport  VectorParamsAs1DForOutWhenUnconnected=off
  wires:
  Logical Operator/1 -> Speed Request/Enable, Bus Creator/1  "ACCEnblReq [Bool]"
  Bus Creator/1 -> Ctrl/1  "ACC"
  Speed Request/1(rpm) -> Bus Creator/2  "ACCSpdReq [rpm]"
  Bus Selector2/1 -> Logical Operator/3  "<ACCReq [Bool]>"
  RelOp(w/Hyst)1/1 -> Logical Operator/5
  Bus Selector1/2 -> Logical Operator1/2  "<RunMode [Bool]>"
  Bus Selector1/1 -> Logical Operator1/1  "<ChgMode [Bool]>"
  Logical Operator1/1 -> Logical Operator/2
  raptor_adjustment/1 -> Logical Operator/1
  raptor_adjustment1/1 -> RelOp(w/Hyst)/2
  Bus Selector3/1 -> RelOp(w/Hyst)/1  "<ACPress [kPa]>"
  RelOp(w/Hyst)/1 -> Logical Operator/4
  Data/1 -> Bus Selector1/1, Bus Selector2/1, Speed Request/1(Data), Bus Selector4/1, Bus Selector3/1
  Bus Selector4/1 -> RelOp(w/Hyst)1/1  "<ACEvapTemp [degC]>"
  raptor_adjustment2/1 -> RelOp(w/Hyst)1/2

== system VCMGCM1962020b_v2/Fgnd/Control/Other/Brake Vacuum Pump ==
  Data : Inport
  Bus Selector : BusSelector  OutputSignals=Control.Mode.StartStop.RunMode [Bool]
  Bus Selector1 : BusSelector  OutputSignals=Sensors.Sensors.Other.BrkVacuumPress.BrkVacuumPress [kPa]
  Header : Blocks_lib/Header  width=Portrait  addtext=''
  Logical Operator : Logic  Inputs=3  OutDataTypeStr=boolean
  RelOp(w/Hyst) : Blocks_lib/RelOp(w//Hyst)  relop=>=
  raptor_adjustment : Raptor_lib/Data Storage/raptor_adjustment  paramName='BrkVacuumPumpEnbl'  nameSource=Parameter  initValue=0  dataType=boolean  storage=Calibration  calDispType=Number  calEnum={'False', 'True'}  calGain=1  calOffset=0  calMax=inf  calMin=-inf  calFormat=''  calUnit='Bool'  calHelp='Brake vacuum pump enable'  calAccess=1  calFunction='Control | Brake Vacuum Pump'  calDispHeaders=off  calColHeaders={'Col1' 'Col2' 'Col3'}  calRowHeaders={'Row1' 'Row2' 'Row3'}
      settings: SourceProductName=Raptor
  raptor_adjustment1 : Raptor_lib/Data Storage/raptor_adjustment  paramName='BrkVacuumPumpThr'  nameSource=Parameter  initValue=[0 0]  dataType=double  storage=Calibration  calDispType=Number  calEnum={'False', 'True'}  calGain=1.0  calOffset=0.0  calMax=inf  calMin=-inf  calFormat=''  calUnit='kPa'  calHelp='Brake vacuum pump threshold (on vacuum pressure)'  calAccess=1  calFunction='Control | Brake Vacuum Pump'  calDispHeaders=off  calColHeaders={'Col1' 'Col2' 'Col3'}  calRowHeaders={'Row1' 'Row2' 'Row3'}
      settings: SourceProductName=Raptor
  Bool : Outport  VectorParamsAs1DForOutWhenUnconnected=off
  wires:
  RelOp(w/Hyst)/1 -> Logical Operator/3
  Bus Selector1/1 -> RelOp(w/Hyst)/1  "<BrkVacuumPress [kPa]>"
  raptor_adjustment1/1 -> RelOp(w/Hyst)/2
  Logical Operator/1 -> Bool/1
  Data/1 -> Bus Selector/1, Bus Selector1/1
  Bus Selector/1 -> Logical Operator/2  "<RunMode [Bool]>"
  raptor_adjustment/1 -> Logical Operator/1

== system VCMGCM1962020b_v2/Fgnd/Control/Other/Cooling Fan ==
  Data : Inport
  Add : Sum  Inputs=+-
  Add1 : Sum  Inputs=+-
  Bus Selector : BusSelector  OutputSignals=Control.Mode.StartStop.ChgMode [Bool],Control.Mode.StartStop.RunMode [Bool]
  Bus Selector1 : BusSelector  OutputSignals=VirtualSensors.Spd.VehSpd [kph]
  Bus Selector2 : BusSelector  OutputSignals=VirtualSensors.Other.CoolTemp1 [degC]
  Bus Selector3 : BusSelector  OutputSignals=VirtualSensors.Other.CoolTemp2 [degC]
  Bus Selector4 : BusSelector  OutputSignals=VirtualSensors.Other.CoolTemp2 [degC],VirtualSensors.Other.AmbientAirTemp [degC]
  Bus Selector5 : BusSelector  OutputSignals=VirtualSensors.Other.CoolTemp1 [degC],VirtualSensors.Other.AmbientAirTemp [degC]
  Bus Selector6 : BusSelector  OutputSignals=VirtualSensors.Other.ACPress [kPa]
  Header : Blocks_lib/Header  width=Portrait  addtext=''
  Logical Operator : Logic  Operator=OR  OutDataTypeStr=boolean
  Logical Operator1 : Logic  Inputs=3  OutDataTypeStr=boolean
  Logical Operator2 : Logic  OutDataTypeStr=boolean
  Logical Operator3 : Logic  Operator=OR  Inputs=3  OutDataTypeStr=boolean
  Logical Operator4 : Logic  OutDataTypeStr=boolean
  Logical Operator5 : Logic  OutDataTypeStr=boolean
  RelOp(w/Hyst) : Blocks_lib/RelOp(w//Hyst)  relop=<=
  RelOp(w/Hyst){1..5} (5 alike) : Blocks_lib/RelOp(w//Hyst)  relop=>=
  raptor_adjustment : Raptor_lib/Data Storage/raptor_adjustment  paramName='CoolFanEnbl'  nameSource=Parameter  initValue=0  dataType=boolean  storage=Calibration  calDispType=Number  calEnum={'False', 'True'}  calGain=1  calOffset=0  calMax=inf  calMin=-inf  calFormat=''  calUnit='Bool'  calHelp='Cooling fan enable'  calAccess=1  calFunction='Control | Cooling Loop'  calDispHeaders=off  calColHeaders={'Col1' 'Col2' 'Col3'}  calRowHeaders={'Row1' 'Row2' 'Row3'}
      settings: SourceProductName=Raptor
  raptor_adjustment1 : Raptor_lib/Data Storage/raptor_adjustment  paramName='CoolFanVehSpdThr'  nameSource=Parameter  initValue=[0 0]  dataType=double  storage=Calibration  calDispType=Number  calEnum={'False', 'True'}  calGain=1.0  calOffset=0.0  calMax=inf  calMin=-inf  calFormat=''  calUnit='kph'  calHelp='Cooling fan threshold (on vehicle speed)'  calAccess=1  calFunction='Control | Cooling Loop'  calDispHeaders=off  calColHeaders={'Col1' 'Col2' 'Col3'}  calRowHeaders={'Row1' 'Row2' 'Row3'}
      settings: SourceProductName=Raptor
  raptor_adjustment2 : Raptor_lib/Data Storage/raptor_adjustment  paramName='CoolFanCoolTemp1Thr'  nameSource=Parameter  initValue=[0 0]  dataType=double  storage=Calibration  calDispType=Number  calEnum={'False', 'True'}  calGain=1.0  calOffset=0.0  calMax=inf  calMin=-inf  calFormat=''  calUnit='degC'  calHelp='Cooling fan threshold (on coolant temperature 1)'  calAccess=1  calFunction='Control | Cooling Loop'  calDispHeaders=off  calColHeaders={'Col1' 'Col2' 'Col3'}  calRowHeaders={'Row1' 'Row2' 'Row3'}
      settings: SourceProductName=Raptor
  raptor_adjustment3 : Raptor_lib/Data Storage/raptor_adjustment  paramName='CoolFanCoolTemp1DeltaThr'  nameSource=Parameter  initValue=[0 0]  dataType=double  storage=Calibration  calDispType=Number  calEnum={'False', 'True'}  calGain=1.0  calOffset=0.0  calMax=inf  calMin=-inf  calFormat=''  calUnit='degC'  calHelp='Cooling fan threshold (on coolant temperature 1 delta over air temperature)'  calAccess=1  calFunction='Control | Cooling Loop'  calDispHeaders=off  calColHeaders={'Col1' 'Col2' 'Col3'}  calRowHeaders={'Row1' 'Row2' 'Row3'}
      settings: SourceProductName=Raptor
  raptor_adjustment4 : Raptor_lib/Data Storage/raptor_adjustment  paramName='CoolFanCoolTemp2Thr'  nameSource=Parameter  initValue=[0 0]  dataType=double  storage=Calibration  calDispType=Number  calEnum={'False', 'True'}  calGain=1.0  calOffset=0.0  calMax=inf  calMin=-inf  calFormat=''  calUnit='degC'  calHelp='Cooling fan threshold (on coolant temperature 2)'  calAccess=1  calFunction='Control | Cooling Loop'  calDispHeaders=off  calColHeaders={'Col1' 'Col2' 'Col3'}  calRowHeaders={'Row1' 'Row2' 'Row3'}
      settings: SourceProductName=Raptor
  raptor_adjustment5 : Raptor_lib/Data Storage/raptor_adjustment  paramName='CoolFanCoolTemp2DeltaThr'  nameSource=Parameter  initValue=[0 0]  dataType=double  storage=Calibration  calDispType=Number  calEnum={'False', 'True'}  calGain=1.0  calOffset=0.0  calMax=inf  calMin=-inf  calFormat=''  calUnit='degC'  calHelp='Cooling fan threshold (on coolant temperature 2 delta over air temperature)'  calAccess=1  calFunction='Control | Cooling Loop'  calDispHeaders=off  calColHeaders={'Col1' 'Col2' 'Col3'}  calRowHeaders={'Row1' 'Row2' 'Row3'}
      settings: SourceProductName=Raptor
  raptor_adjustment6 : Raptor_lib/Data Storage/raptor_adjustment  paramName='CoolFanACPressThr'  nameSource=Parameter  initValue=[0 0]  dataType=double  storage=Calibration  calDispType=Number  calEnum={'False', 'True'}  calGain=1.0  calOffset=0.0  calMax=inf  calMin=-inf  calFormat=''  calUnit='kPa'  calHelp='Cooling fan threshold (on A/C pressure)'  calAccess=1  calFunction='Control | Cooling Loop'  calDispHeaders=off  calColHeaders={'Col1' 'Col2' 'Col3'}  calRowHeaders={'Row1' 'Row2' 'Row3'}
      settings: SourceProductName=Raptor
  Bool : Outport  VectorParamsAs1DForOutWhenUnconnected=off
  wires:
  Logical Operator2/1 -> Bool/1
  Bus Selector/1 -> Logical Operator/1  "<ChgMode [Bool]>"
  Bus Selector/2 -> Logical Operator/2  "<RunMode [Bool]>"
  Bus Selector4/1 -> Add1/1  "<CoolTemp2 [degC]>"
  Logical Operator3/1 -> Logical Operator2/2
  RelOp(w/Hyst)2/1 -> Logical Operator4/2
  RelOp(w/Hyst)5/1 -> Logical Operator3/3
  Add1/1 -> RelOp(w/Hyst)4/1
  RelOp(w/Hyst)3/1 -> Logical Operator5/1
  Bus Selector4/2 -> Add1/2  "<AmbientAirTemp [degC]>"
  Bus Selector5/1 -> Add/1  "<CoolTemp1 [degC]>"
  Data/1 -> Bus Selector1/1, Bus Selector2/1, Bus Selector3/1, Bus Selector4/1, Bus Selector6/1, Bus Selector5/1, Bus Selector/1
  Add/1 -> RelOp(w/Hyst)2/1
  Logical Operator5/1 -> Logical Operator3/2
  Bus Selector3/1 -> RelOp(w/Hyst)3/1  "<CoolTemp2 [degC]>"
  Bus Selector2/1 -> RelOp(w/Hyst)1/1  "<CoolTemp1 [degC]>"
  raptor_adjustment5/1 -> RelOp(w/Hyst)4/2
  raptor_adjustment1/1 -> RelOp(w/Hyst)/2
  Bus Selector1/1 -> RelOp(w/Hyst)/1  "<VehSpd [kph]>"
  raptor_adjustment6/1 -> RelOp(w/Hyst)5/2
  Bus Selector6/1 -> RelOp(w/Hyst)5/1  "<ACPress [kPa]>"
  Bus Selector5/2 -> Add/2  "<AmbientAirTemp [degC]>"
  raptor_adjustment3/1 -> RelOp(w/Hyst)2/2
  RelOp(w/Hyst)4/1 -> Logical Operator5/2
  raptor_adjustment4/1 -> RelOp(w/Hyst)3/2
  raptor_adjustment2/1 -> RelOp(w/Hyst)1/2
  RelOp(w/Hyst)1/1 -> Logical Operator4/1
  Logical Operator4/1 -> Logical Operator3/1
  raptor_adjustment/1 -> Logical Operator1/1
  Logical Operator/1 -> Logical Operator1/2
  RelOp(w/Hyst)/1 -> Logical Operator1/3
  Logical Operator1/1 -> Logical Operator2/1
